simulink model "modelo_accionamiento_izaje"  (R2023a)
settings: Solver=ode15s  StartTime=0.0  StopTime=100  RelTol=1e-3
InitFcn:
  | parametros
  | gain_CL
values from neighbouring files (symbols this model uses):
  b_cy = 1e7    (= 10000000)    [parametros.m]
  b_ha = -(J_hEq + (r_hd/(2*i_h))*m_l) * w_des_h*(1 + n_h + n_h^2) + b_hEq    [gain_CL.m]
  b_hd = 8    [parametros.m]
  b_hm = 18    [parametros.m]
  b_wu = 150    [parametros.m]
  g = 9.80664    [parametros.m]
  i_h = 22    [parametros.m]
  J_hd_hEb = 3800    [parametros.m]
  J_hm_hb = 30    [parametros.m]
  K_cy = 1.8e9    (= 1800000000)    [parametros.m]
  k_hsa = -(J_hEq + (r_hd/(2*i_h))*m_l) * w_des_h^2*(n_h + n_h^2 + n_h^3)    [gain_CL.m]
  k_hsia = -(J_hEq + (r_hd/(2*i_h))*m_l) * n_h^3 * w_des_h^3    [gain_CL.m]
  k_wu = 2.36e8    (= 236000000)    [parametros.m]
  m_l = M_s+M_cmax    (= 65000)    [parametros.m]
  r_hd = 0.75    [parametros.m]
  theta_hm0 = -l_h0*i_h*2/r_hd    (= -293.333333333)    [parametros.m]
  v_lx0 = 0    [parametros.m]
  v_ly0 = 0    [parametros.m]
  w_hm0 = 0    [parametros.m]
  x_l0 = 0    [parametros.m]
  y_l0 = 40    [parametros.m]
  Y_t0 = 45    [parametros.m]
libraries: simulink x8
settings Model: Creator=Usuario  LastModifiedBy=Usuario

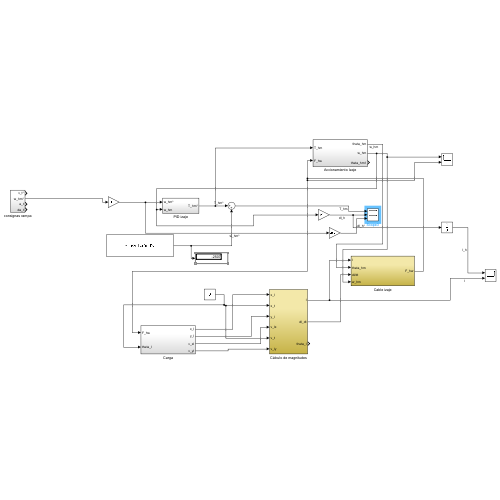
[thumbnail: Simulink's stored preview of the top-level diagram]
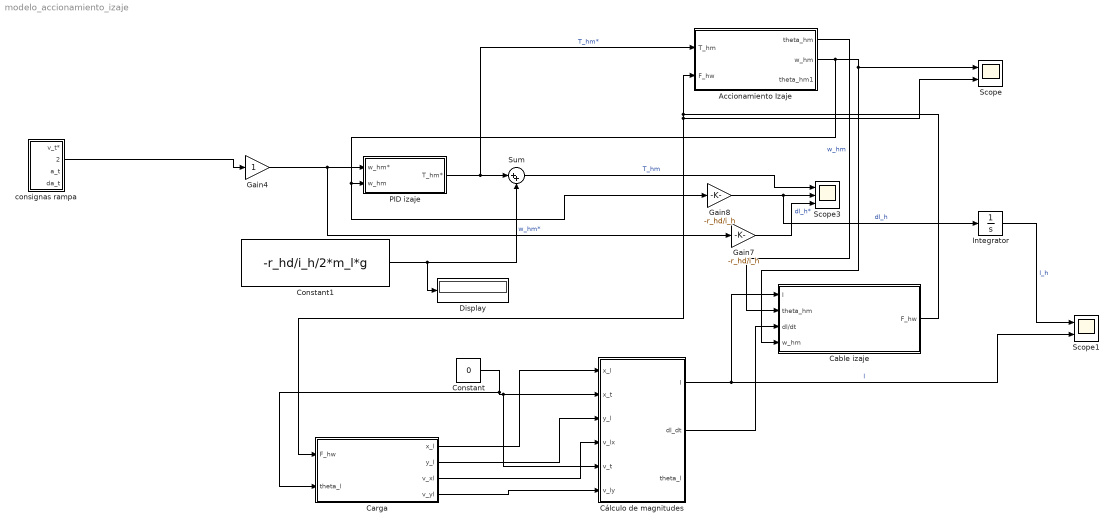
== system modelo_accionamiento_izaje ==
  Accionamiento Izaje : Subsystem
  Cable izaje : Subsystem
  Carga : Subsystem
  Constant : Constant  Value=0
  Constant1 : Constant  Value=-r_hd/i_h/2*m_l*g
  Cálculo de magnitudes : Subsystem
  Display : Display
  Gain4 : Gain
  Gain7 : Gain  Gain=-r_hd/i_h
  Gain8 : Gain  Gain=-r_hd/i_h
  Integrator : Integrator
  PID izaje : Subsystem
  Scope : Scope  NumInputPorts=2
  Scope1 : Scope  NumInputPorts=2
  Scope3 : Scope  NumInputPorts=3
  Sum : Sum  Inputs=|++
  consignas rampa : Subsystem
  wires:
  Gain7/1 -> Scope3/3  "dl_h*"
  consignas rampa/2(w_hm*) -> Gain4/1
  Gain4/1 -> Gain7/1, PID izaje/1(w_hm*)  "w_hm*"
  Gain8/1 -> Integrator/1, Scope3/2  "dl_h"
  PID izaje/1(T_hm*) -> Sum/1, Accionamiento Izaje/1(T_hm)  "T_hm*"
  Cálculo de magnitudes/1(l) -> Scope1/2, Cable izaje/1(l)  "l"
  Cálculo de magnitudes/2(dl_dt) -> Cable izaje/3(dl/dt)
  Carga/1(x_l) -> Cálculo de magnitudes/1(x_l)
  Constant/1 -> Carga/2(theta_l), Cálculo de magnitudes/5(v_t), Cálculo de magnitudes/2(x_t)
  Carga/2(y_l) -> Cálculo de magnitudes/3(y_l)
  Carga/3(v_xl) -> Cálculo de magnitudes/4(v_lx)
  Carga/4(v_yl) -> Cálculo de magnitudes/6(v_ly)
  Accionamiento Izaje/2(w_hm) -> Gain8/1, PID izaje/2(w_hm), Cable izaje/4(w_hm), Scope/1
  Cable izaje/1(F_hw) -> Scope/2, Carga/1(F_hw), Accionamiento Izaje/2(F_hw)
  Accionamiento Izaje/1(theta_hm) -> Cable izaje/2(theta_hm)  "w_hm"
  Sum/1 -> Scope3/1  "T_hm"
  Constant1/1 -> Display/1, Sum/2
  Integrator/1 -> Scope1/1  "l_h"

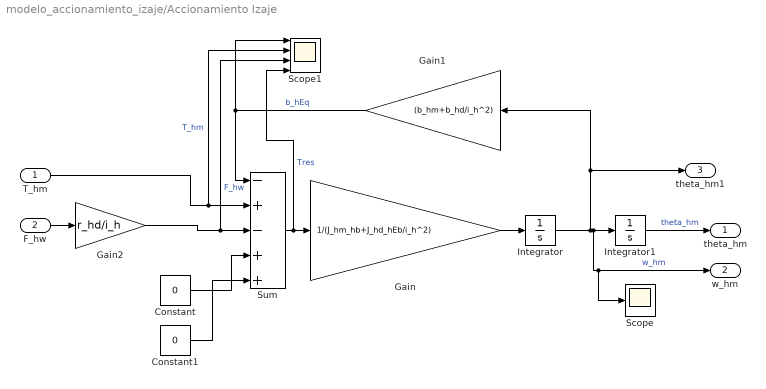
== system modelo_accionamiento_izaje/Accionamiento Izaje ==
  T_hm : Inport
  F_hw : Inport  Port=2
  Constant : Constant  Value=0
  Constant1 : Constant  Value=0
  Gain : Gain  Gain=1/(J_hm_hb+J_hd_hEb/i_h^2)
  Gain1 : Gain  Gain=(b_hm+b_hd/i_h^2)
  Gain2 : Gain  Gain=r_hd/i_h
  Integrator : Integrator  InitialCondition=w_hm0
  Integrator1 : Integrator  InitialCondition=theta_hm0
  Scope : Scope
  Scope1 : Scope  NumInputPorts=4
  Sum : Sum  Inputs=-+-++
  theta_hm : Outport
  w_hm : Outport  Port=2
  theta_hm1 : Outport  Port=3
  wires:
  Integrator1/1 -> theta_hm/1  "theta_hm"
  Integrator/1 -> Gain1/1, theta_hm1/1, Scope/1, w_hm/1, Integrator1/1  "w_hm"
  Gain/1 -> Integrator/1
  Sum/1 -> Scope1/4, Gain/1  "Tres"
  Gain1/1 -> Sum/1, Scope1/1  "b_hEq"
  F_hw/1 -> Gain2/1
  Constant1/1 -> Sum/5
  Gain2/1 -> Scope1/3, Sum/3  "F_hw"
  T_hm/1 -> Scope1/2, Sum/2  "T_hm"
  Constant/1 -> Sum/4

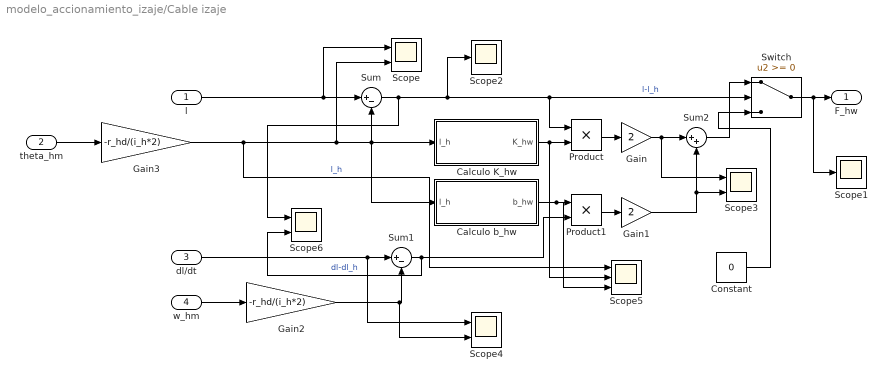
== system modelo_accionamiento_izaje/Cable izaje ==
  l : Inport
  theta_hm : Inport  Port=2
  dl/dt : Inport  Port=3
  w_hm : Inport  Port=4
  Calculo K_hw : Subsystem
  Calculo b_hw : Subsystem
  Constant : Constant  Value=0
  Gain : Gain  Gain=2
  Gain1 : Gain  Gain=2
  Gain2 : Gain  Gain=-r_hd/(i_h*2)
  Gain3 : Gain  Gain=-r_hd/(i_h*2)
  Product : Product
  Product1 : Product
  Scope{,3..4,6} (4 alike) : Scope  NumInputPorts=2
  Scope1 : Scope
  Scope2 : Scope
  Scope5 : Scope  NumInputPorts=3
  Sum : Sum  Inputs=|+-
  Sum1 : Sum  Inputs=|+-
  Sum2 : Sum  Inputs=|++
  Switch : Switch  SaturateOnIntegerOverflow=off  InputSameDT=off
  F_hw : Outport
  wires:
  l/1 -> Scope/1, Sum/1
  theta_hm/1 -> Gain3/1
  Sum/1 -> Scope6/1, Scope2/1, Product/1, Switch/2  "l-l_h"
  Calculo K_hw/1(K_hw) -> Scope5/2, Product/2
  Product/1 -> Gain/1
  w_hm/1 -> Gain2/1
  Product1/1 -> Gain1/1
  Calculo b_hw/1(b_hw) -> Scope5/3, Product1/1
  Gain1/1 -> Scope3/2, Sum2/2
  Gain/1 -> Scope3/1, Sum2/1
  Sum2/1 -> Switch/1
  Switch/1 -> Scope1/1, F_hw/1
  dl/dt/1 -> Scope4/1, Sum1/1
  Constant/1 -> Switch/3
  Gain2/1 -> Scope4/2, Sum1/2
  Gain3/1 -> Scope5/1, Calculo b_hw/1(l_h), Calculo K_hw/1(l_h), Sum/2, Scope/2  "l_h"
  Sum1/1 -> Scope6/2, Product1/2  "dl-dl_h"

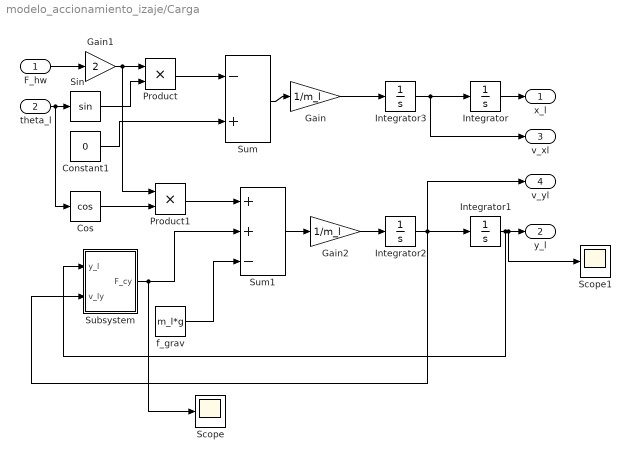
== system modelo_accionamiento_izaje/Carga ==
  F_hw : Inport
  theta_l : Inport  Port=2
  Constant1 : Constant  Value=0
  Cos : Trigonometry  Operator=cos
  Gain : Gain  Gain=1/m_l
  Gain1 : Gain  Gain=2
  Gain2 : Gain  Gain=1/m_l
  Integrator : Integrator  InitialCondition=x_l0
  Integrator1 : Integrator  InitialCondition=y_l0
  Integrator2 : Integrator  InitialCondition=v_ly0
  Integrator3 : Integrator  InitialCondition=v_lx0
  Product : Product
  Product1 : Product
  Scope : Scope
  Scope1 : Scope
  Sin : Trigonometry
  Subsystem : Subsystem
  Sum : Sum  Inputs=-+
  Sum1 : Sum  Inputs=++-
  f_grav : Constant  Value=m_l*g
  x_l : Outport
  y_l : Outport  Port=2
  v_xl : Outport  Port=3
  v_yl : Outport  Port=4
  wires:
  Sum/1 -> Gain/1
  Gain/1 -> Integrator3/1
  theta_l/1 -> Cos/1, Sin/1
  F_hw/1 -> Gain1/1
  Gain1/1 -> Product/1, Product1/1
  Sin/1 -> Product/2
  Product/1 -> Sum/1
  Constant1/1 -> Sum/2
  Product1/1 -> Sum1/1
  Cos/1 -> Product1/2
  f_grav/1 -> Sum1/3
  Subsystem/1(F_cy) -> Scope/1, Sum1/2
  Gain2/1 -> Integrator2/1
  Sum1/1 -> Gain2/1
  Integrator/1 -> x_l/1
  Integrator3/1 -> v_xl/1, Integrator/1
  Integrator2/1 -> v_yl/1, Subsystem/2(v_ly), Integrator1/1
  Integrator1/1 -> Subsystem/1(y_l), Scope1/1, y_l/1

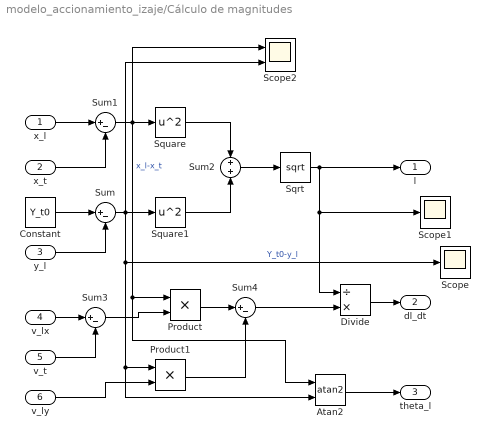
== system modelo_accionamiento_izaje/Cálculo de magnitudes ==
  x_l : Inport
  x_t : Inport  Port=2
  y_l : Inport  Port=3
  v_lx : Inport  Port=4
  v_t : Inport  Port=5
  v_ly : Inport  Port=6
  Atan2 : Trigonometry  Operator=atan2
  Constant : Constant  Value=Y_t0
  Divide : Product  Inputs=/*
  Product : Product
  Product1 : Product
  Scope : Scope
  Scope1 : Scope
  Scope2 : Scope  NumInputPorts=2
  Sqrt : Sqrt
  Square : Math  Operator=square
  Square1 : Math  Operator=square
  Sum{,1,3..4} (4 alike) : Sum  Inputs=|+-
  Sum2 : Sum  Inputs=+|+
  l : Outport
  dl_dt : Outport  Port=2
  theta_l : Outport  Port=3
  wires:
  Constant/1 -> Sum/1
  y_l/1 -> Sum/2
  x_l/1 -> Sum1/1
  x_t/1 -> Sum1/2
  Sum1/1 -> Scope2/1, Atan2/1, Product/1, Square/1  "x_l-x_t"
  Sum/1 -> Scope2/2, Atan2/2, Product1/1, Scope/1, Square1/1  "Y_t0-y_l"
  Square/1 -> Sum2/1
  Square1/1 -> Sum2/2
  Sum2/1 -> Sqrt/1
  Sqrt/1 -> Divide/1, Scope1/1, l/1
  v_lx/1 -> Sum3/1
  v_t/1 -> Sum3/2
  Sum3/1 -> Product/2
  Product/1 -> Sum4/1
  v_ly/1 -> Product1/2
  Product1/1 -> Sum4/2
  Sum4/1 -> Divide/2
  Divide/1 -> dl_dt/1
  Atan2/1 -> theta_l/1

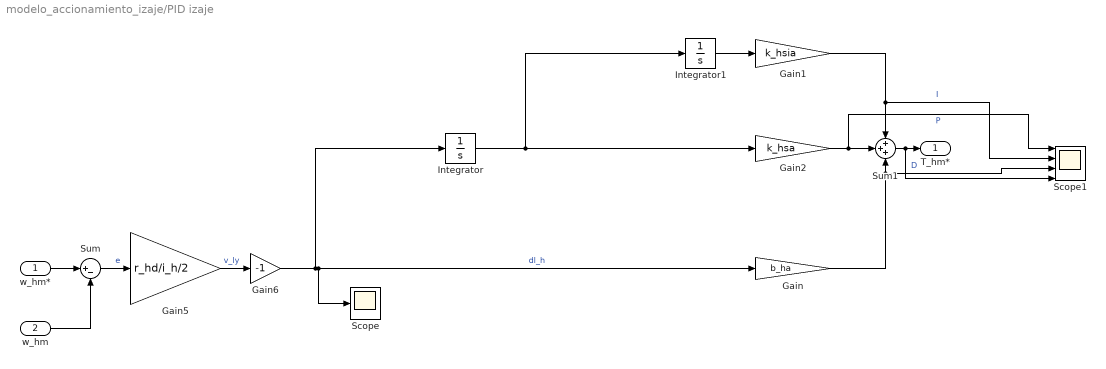
== system modelo_accionamiento_izaje/PID izaje ==
  w_hm* : Inport
  w_hm : Inport  Port=2
  Gain : Gain  Gain=b_ha
  Gain1 : Gain  Gain=k_hsia
  Gain2 : Gain  Gain=k_hsa
  Gain5 : Gain  Gain=r_hd/i_h/2
  Gain6 : Gain  Gain=-1
  Integrator : Integrator
  Integrator1 : Integrator
  Scope : Scope
  Scope1 : Scope  NumInputPorts=4
  Sum : Sum  Inputs=|+-
  Sum1 : Sum  Inputs=+++
  T_hm* : Outport
  wires:
  Gain2/1 -> Scope1/1, Sum1/2  "P"
  w_hm*/1 -> Sum/1
  Gain/1 -> Scope1/3, Sum1/3  "D"
  Gain1/1 -> Scope1/2, Sum1/1  "I"
  w_hm/1 -> Sum/2
  Sum1/1 -> Scope1/4, T_hm*/1
  Sum/1 -> Gain5/1  "e"
  Gain5/1 -> Gain6/1  "v_ly"
  Gain6/1 -> Integrator/1, Scope/1, Gain/1  "dl_h"
  Integrator/1 -> Integrator1/1, Gain2/1
  Integrator1/1 -> Gain1/1

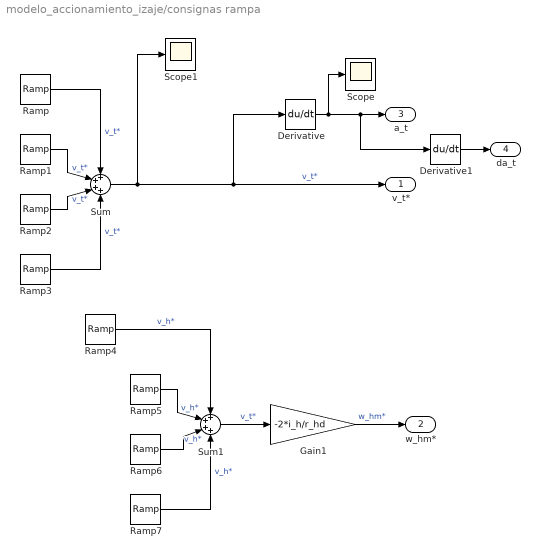
== system modelo_accionamiento_izaje/consignas rampa ==
  Derivative : Derivative
  Derivative1 : Derivative
  Gain1 : Gain  Gain=-2*i_h/r_hd
  Ramp : simulink/Sources/Ramp  slope=0.8  start=5  InitialOutput=0
  Ramp1 : simulink/Sources/Ramp  slope=-0.8  start=10  InitialOutput=0
  Ramp2 : simulink/Sources/Ramp  slope=-0.8  start=35  InitialOutput=0
  Ramp3 : simulink/Sources/Ramp  slope=0.8  start=40  InitialOutput=0
  Ramp4 : simulink/Sources/Ramp  slope=2  start=5  InitialOutput=0
  Ramp5 : simulink/Sources/Ramp  slope=-2  start=9  InitialOutput=0
  Ramp6 : simulink/Sources/Ramp  slope=-2  start=15  InitialOutput=0
  Ramp7 : simulink/Sources/Ramp  slope=2  start=19  InitialOutput=0
  Scope : Scope
  Scope1 : Scope
  Sum : Sum  Inputs=++++
  Sum1 : Sum  Inputs=++++
  v_t* : Outport
  w_hm* : Outport  Port=2
  a_t : Outport  Port=3
  da_t : Outport  Port=4
  wires:
  Ramp3/1 -> Sum/4  "v_t*"
  Sum/1 -> Scope1/1, v_t*/1, Derivative/1  "v_t*"
  Ramp1/1 -> Sum/2  "v_t*"
  Ramp/1 -> Sum/1  "v_t*"
  Ramp2/1 -> Sum/3  "v_t*"
  Ramp6/1 -> Sum1/3  "v_h*"
  Sum1/1 -> Gain1/1  "v_t*"
  Ramp5/1 -> Sum1/2  "v_h*"
  Ramp4/1 -> Sum1/1  "v_h*"
  Ramp7/1 -> Sum1/4  "v_h*"
  Gain1/1 -> w_hm*/1  "w_hm*"
  Derivative/1 -> Scope/1, Derivative1/1, a_t/1
  Derivative1/1 -> da_t/1

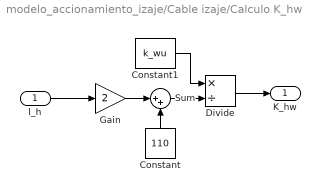
== system modelo_accionamiento_izaje/Cable izaje/Calculo K_hw ==
  l_h : Inport
  Constant : Constant  Value=110
  Constant1 : Constant  Value=k_wu
  Divide : Product  Inputs=*/
  Gain : Gain  Gain=2
  Sum : Sum  Inputs=|++
  K_hw : Outport
  wires:
  l_h/1 -> Gain/1
  Gain/1 -> Sum/1
  Constant/1 -> Sum/2
  Sum/1 -> Divide/2
  Constant1/1 -> Divide/1
  Divide/1 -> K_hw/1

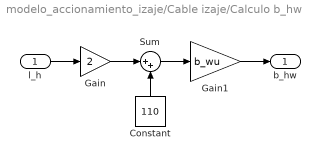
== system modelo_accionamiento_izaje/Cable izaje/Calculo b_hw ==
  l_h : Inport
  Constant : Constant  Value=110
  Gain : Gain  Gain=2
  Gain1 : Gain  Gain=b_wu
  Sum : Sum  Inputs=|++
  b_hw : Outport
  wires:
  l_h/1 -> Gain/1
  Gain/1 -> Sum/1
  Constant/1 -> Sum/2
  Sum/1 -> Gain1/1
  Gain1/1 -> b_hw/1

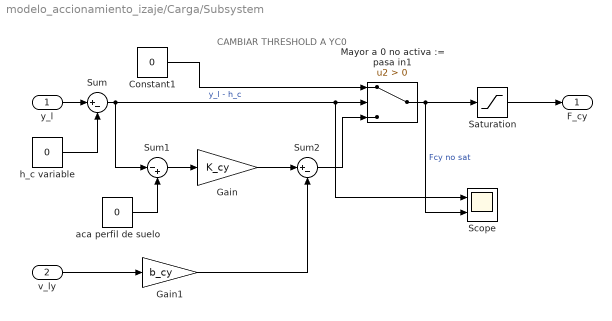
== system modelo_accionamiento_izaje/Carga/Subsystem ==
  note: CAMBIAR THRESHOLD A YC0
  y_l : Inport
  v_ly : Inport  Port=2
  Constant1 : Constant  Value=0
  Gain : Gain  Gain=K_cy
  Gain1 : Gain  Gain=b_cy
  Mayor a 0 no activa := pasa in1 : Switch  Criteria=u2 > Threshold  SaturateOnIntegerOverflow=off  InputSameDT=off
  Saturation : Saturate  UpperLimit=inf  LowerLimit=0
  Scope : Scope  NumInputPorts=2
  Sum : Sum  Inputs=|+-
  Sum1 : Sum  Inputs=|-+
  Sum2 : Sum  Inputs=|+-
  aca perfil de suelo : Constant  Value=0
  h_c variable : Constant  Value=0
  F_cy : Outport
  wires:
  Mayor a 0 no activa := pasa in1/1 -> Scope/2, Saturation/1  "Fcy no sat"
  Sum2/1 -> Mayor a 0 no activa := pasa in1/3
  Constant1/1 -> Mayor a 0 no activa := pasa in1/1
  Sum/1 -> Sum1/1, Scope/1, Mayor a 0 no activa := pasa in1/2  "y_l - h_c"
  y_l/1 -> Sum/1
  h_c variable/1 -> Sum/2
  aca perfil de suelo/1 -> Sum1/2
  Sum1/1 -> Gain/1
  Gain/1 -> Sum2/1
  v_ly/1 -> Gain1/1
  Gain1/1 -> Sum2/2
  Saturation/1 -> F_cy/1
